simulink model "MCHP_SMO_MCLV48V300W_dsPIC33CK256MP508_DIM"  (R2022b)
settings: Solver=FixedStepDiscrete  StartTime=0.0  StopTime=10.0  FixedStep=50e-6  RelTol=1e-3  EnableMultiTasking=on
values from neighbouring files (symbols this model uses):
  Iq_Ref_openLoop = 1.5    [mcb_pmsm_foc_SMO_dsPIC33_data.m]
  PI_params = mcb.internal.SetControllerParameters(pmsm,inverter,PU_System,T_pwm,Ts,Ts_speed)    [mcb_pmsm_foc_SMO_dsPIC33_data.m]
  PU_System = mcb_SetPUSystem(pmsm,inverter)    [mcb_pmsm_foc_SMO_dsPIC33_data.m]
  PWM_frequency = 20e3    (= 20000)    [mcb_pmsm_foc_SMO_dsPIC33_data.m]
  Speed_Ref_openLoop = 700    [mcb_pmsm_foc_SMO_dsPIC33_data.m]
  Ts = T_pwm    (= 5e-05)    [mcb_pmsm_foc_SMO_dsPIC33_data.m]
  Ts_speed = 30*Ts    (= 0.0015)    [mcb_pmsm_foc_SMO_dsPIC33_data.m]
undefined symbols (not defined in the file or in its folder): A0, A4, AN0, AN1, B0, B2, C10, C11, C4, C5, D13, D14, D2, DiscIntNeverNeededParam, inverter, Max, MaxPer, ms, NumBits1, NumBits2, P20, P32, P52, P53, P58, P59, P66, P77, P78, Pin, pmsm, PWM1max, Resol, s, us
libraries: simulink x30, MCHP_Blockset x19, mcbcontrolslib x9, slpidlib x3, mcbplantlib x1, autolibpmsmexterior x1
(part 4 of 4)

== system MCHP_SMO_MCLV48V300W_dsPIC33CK256MP508_DIM/Current Control/Position and Speed Estimation1/Openloop Pos_PU ==
  Reset : ResetPort  DisableCoverage=on
  Constant : Constant  Value=Speed_Ref_openLoop/PU_System.N_base  OutDataTypeStr=dataType
  Data Type Conversion : DataTypeConversion  OutDataTypeStr=fixdt(1,32,20)  ConvertRealWorld=Stored Integer (SI)  SaturateOnIntegerOverflow=off  RndMeth=Floor
  Discrete-Time Integrator : DiscreteIntegrator  IntegratorMethod=Accumulation: Forward Euler  gainval=0.002  SampleTime=Ts  OutDataTypeStr=fixdt(1,32,20)  LimitOutput=on  UpperSaturationLimit=Speed_Ref_openLoop/PU_System.N_base  LowerSaturationLimit=0  ICPrevOutput=DiscIntNeverNeededParam  ICPrevScaledInput=DiscIntNeverNeededParam
  Gain : Gain  Gain=Ts*PU_System.N_base*pmsm.p/60  OutDataTypeStr=dataType  ParamDataTypeStr=Inherit: Same as input
  Position Generator : mcbcontrolslib/Position Generator  AngleOutput=Per-unit  ThetaSource=External  ThetaInput=5e-4  DataType=double  ExternalReset=none  Offset=0
  eps : Outport
  wires:
  Constant/1 -> Data Type Conversion/1
  Data Type Conversion/1 -> Discrete-Time Integrator/1
  Discrete-Time Integrator/1 -> Gain/1
  Position Generator/1 -> eps/1
  Gain/1 -> Position Generator/1

== system MCHP_SMO_MCLV48V300W_dsPIC33CK256MP508_DIM/Current Control/Position and Speed Estimation1/OpentoClosed ==
  Speed_fb : Inport
  Chart : Stateflow chart  TreatAsAtomicUnit=on
  Data Store Read5 : DataStoreRead  DataStoreName=Enable  IndexOptions=Index vector (dialog)  Indices=1  OutputSizes=1
  Data Store Write2 : DataStoreWrite  DataStoreName=EnableClosedLoop  IndexOptions=Index vector (dialog)  Indices=1  OutputSizes=1
  Data Type Conversion : DataTypeConversion  OutDataTypeStr=boolean  RndMeth=Simplest  SaturateOnIntegerOverflow=off
  Enable Closed Loop : Constant  OutDataTypeStr=uint16
  Enable Closed Loop1 : Constant  Value=Speed_Ref_openLoop/PU_System.N_base  OutDataTypeStr=dataType
  Open Loop Start-up : Constant  Value=0  OutDataTypeStr=uint16
  Switch2 : Switch  Criteria=u2 > Threshold  Threshold=1  SaturateOnIntegerOverflow=off  InputSameDT=off
  Terminator : Terminator
  EnClosedLoop : Outport
  wires:
  Open Loop Start-up/1 -> Switch2/3
  Data Store Read5/1 -> Chart/3(En)
  Chart/1(Mode) -> Switch2/2
  Switch2/1 -> Data Type Conversion/1
  Speed_fb/1 -> Chart/2(SpeedFb)
  Enable Closed Loop/1 -> Switch2/1
  Enable Closed Loop1/1 -> Chart/1(Limit)
  Chart/2(SpeedCtrl) -> Terminator/1
  Data Type Conversion/1 -> EnClosedLoop/1, Data Store Write2/1

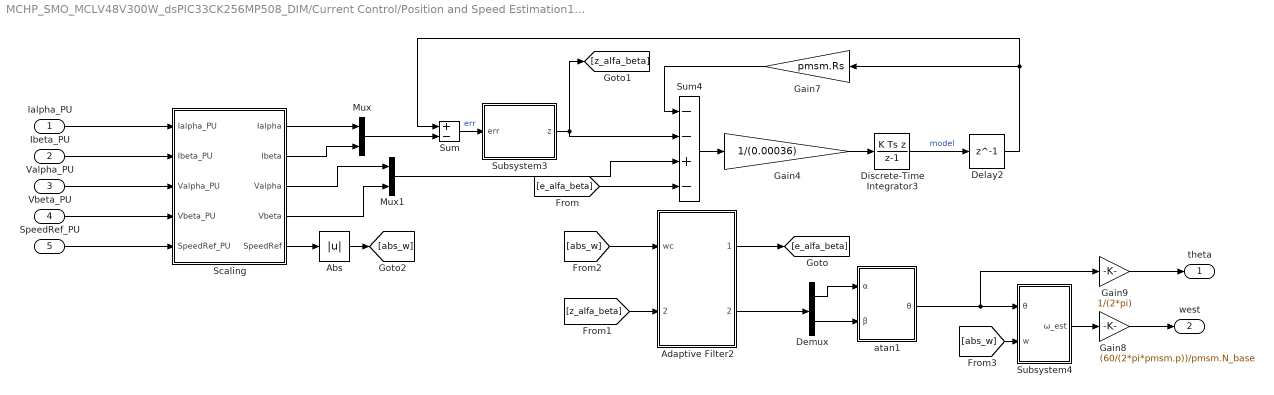
== system MCHP_SMO_MCLV48V300W_dsPIC33CK256MP508_DIM/Current Control/Position and Speed Estimation1/Sliding Mode Observer1 ==
  Ialpha_PU : Inport
  Ibeta_PU : Inport  Port=2
  Valpha_PU : Inport  Port=3
  Vbeta_PU : Inport  Port=4
  SpeedRef_PU : Inport  Port=5
  Abs : Abs  SaturateOnIntegerOverflow=off
  Adaptive Filter2 : Subsystem
  Delay2 : Delay  DelayLength=1
  Demux : Demux  Outputs=2
  Discrete-Time Integrator3 : DiscreteIntegrator  IntegratorMethod=Integration: Backward Euler  SampleTime=-1  OutDataTypeStr=Typecast_ci  ICPrevOutput=DiscIntNeverNeededParam  ICPrevScaledInput=DiscIntNeverNeededParam
  Gain4 : Gain  Gain=1/(0.00036)  OutDataTypeStr=fixdt(1,32,11)
  Gain7 : Gain  Gain=pmsm.Rs  OutDataTypeStr=Inherit: Same as input
  Gain8 : Gain  Gain=(60/(2*pi*pmsm.p))/pmsm.N_base  OutDataTypeStr=dataType
  Gain9 : Gain  Gain=1/(2*pi)  OutDataTypeStr=dataType
  Mux : Mux  Inputs=2
  Mux1 : Mux  Inputs=2
  Scaling : Subsystem
  Subsystem3 : Subsystem
  Subsystem4 : Subsystem
  Sum : Sum  Inputs=+-  AccumDataTypeStr=Typecast_ci  OutDataTypeStr=Typecast_ci
  Sum4 : Sum  Inputs=--+-  AccumDataTypeStr=Typecast_di  OutDataTypeStr=Typecast_di
  atan1 : Subsystem
  theta : Outport
  west : Outport  Port=2
  wires:
  Ialpha_PU/1 -> Scaling/1(Ialpha_PU)
  Vbeta_PU/1 -> Scaling/4(Vbeta_PU)
  Valpha_PU/1 -> Scaling/3(Valpha_PU)
  Ibeta_PU/1 -> Scaling/2(Ibeta_PU)
  SpeedRef_PU/1 -> Scaling/5(SpeedRef_PU)
  Gain7/1 -> Sum4/1
  Discrete-Time Integrator3/1 -> Delay2/1  "model"
  atan1/1(θ) -> Gain9/1, Subsystem4/1(θ)
  Sum4/1 -> Gain4/1
  Mux1/1 -> Sum4/3
  Gain4/1 -> Discrete-Time Integrator3/1
  Subsystem4/1(ω_est) -> Gain8/1
  Subsystem3/1(z) -> [z_alfa_beta], Sum4/2
  Gain9/1 -> theta/1
  Gain8/1 -> west/1
  Sum/1 -> Subsystem3/1(err)  "err"
  Scaling/5(SpeedRef) -> Abs/1
  Scaling/1(Ialpha) -> Mux/1
  Scaling/2(Ibeta) -> Mux/2
  Scaling/3(Valpha) -> Mux1/1
  Scaling/4(Vbeta) -> Mux1/2
  [e_alfa_beta] -> Sum4/4
  Mux/1 -> Sum/2
  Delay2/1 -> Sum/1, Gain7/1
  Adaptive Filter2/1(ealfa_bita) -> [e_alfa_beta]
  Adaptive Filter2/2(ealfa_bita_fil) -> Demux/1
  [z_alfa_beta] -> Adaptive Filter2/2(zalfa_bita)
  Abs/1 -> [abs_w]
  [abs_w] -> Adaptive Filter2/1(wc)
  Demux/1 -> atan1/1(α)
  Demux/2 -> atan1/2(β)
  [abs_w] -> Subsystem4/2(w)

== system MCHP_SMO_MCLV48V300W_dsPIC33CK256MP508_DIM/Current Control/Serial Tx/UART_TX ==
  Count : Inport
  Data : Inport  Port=2
  Debug_Data : Subsystem
  SCI_Tx : Subsystem
  wires:
  Count/1 -> Debug_Data/1(Count)
  Debug_Data/1(Data_log) -> SCI_Tx/1(Data_Log)
  Data/1 -> Debug_Data/2(Data)

== system MCHP_SMO_MCLV48V300W_dsPIC33CK256MP508_DIM/Inverter and Motor/Simulation/Inverter ==
  Duty_abc : Inport
  Average-Value Inverter : mcbplantlib/Average-Value Inverter
  Constant2 : Constant  Value=inverter.V_dc  OutDataTypeStr=single  SampleTime=-1
  Data Type Conversion1 : DataTypeConversion  OutDataTypeStr=single  RndMeth=Simplest  SaturateOnIntegerOverflow=off
  Vabc : Outport  VectorParamsAs1DForOutWhenUnconnected=off
  wires:
  Average-Value Inverter/1 -> Vabc/1
  Data Type Conversion1/1 -> Average-Value Inverter/1
  Duty_abc/1 -> Data Type Conversion1/1
  Constant2/1 -> Average-Value Inverter/2

== system MCHP_SMO_MCLV48V300W_dsPIC33CK256MP508_DIM/Inverter and Motor/Simulation/Load_Profile (Torque) ==
  Data Type Conversion : DataTypeConversion  OutDataTypeStr=single  SaturateOnIntegerOverflow=off  RndMeth=Floor
  IIR Filter : mcbcontrolslib/IIR Filter  VariantControl=Low Pass Filter  VariantSelect=Low-pass  Filter_constant=0.01  advancedSettings=off  Ts=50e-6  cutOff_freq=32.1525
  Rate Limiter1 : RateLimiter  RisingSlewLimit=0.5  FallingSlewLimit=-0.2  SampleTimeMode=inherited
  Step : Step  Time=5  Before=0.0* pmsm.T_rated  After=0.25* pmsm.T_rated
  Step1 : Step  Time=8  Before=0.25* pmsm.T_rated  After=0.7*pmsm.T_rated
  Step2 : Step  Time=8  Before=1  After=0
  Switch : Switch  Criteria=u2 > Threshold  SaturateOnIntegerOverflow=off  InputSameDT=off
  Load_Trq : Outport  VectorParamsAs1DForOutWhenUnconnected=off
  wires:
  IIR Filter/1 -> Load_Trq/1
  Data Type Conversion/1 -> IIR Filter/1
  Switch/1 -> Rate Limiter1/1
  Step1/1 -> Switch/3
  Step/1 -> Switch/1
  Step2/1 -> Switch/2
  Rate Limiter1/1 -> Data Type Conversion/1

== system MCHP_SMO_MCLV48V300W_dsPIC33CK256MP508_DIM/Inverter and Motor/Simulation/Sensor_Measurements ==
  PhaseCurr : Inport
  Data Type Conversion4 : DataTypeConversion  OutDataTypeStr=single  RndMeth=Simplest  SaturateOnIntegerOverflow=off
  Delay1 : Delay  DelayLength=PI_params.delay_Currents
  Inverting OpAmp : Gain  Gain=1/PU_System.I_base  OutDataTypeStr=dataType  RndMeth=Simplest
  Selector : Selector  InputPortWidth=3  IndexOptions=Index vector (dialog)  Indices=[1 2]  OutputSizes=1
  Iab_fb : Outport  VectorParamsAs1DForOutWhenUnconnected=off
  wires:
  Selector/1 -> Inverting OpAmp/1
  PhaseCurr/1 -> Data Type Conversion4/1
  Data Type Conversion4/1 -> Delay1/1
  Delay1/1 -> Selector/1  "Iab_fb"
  Inverting OpAmp/1 -> Iab_fb/1

== system MCHP_SMO_MCLV48V300W_dsPIC33CK256MP508_DIM/Speed Control/Enable Switch/Codegen ==

== system MCHP_SMO_MCLV48V300W_dsPIC33CK256MP508_DIM/Speed Control/Enable Switch/Sim ==
  Constant : Constant  OutDataTypeStr=Inherit: Inherit via back propagation
  Data Store Write : DataStoreWrite  DataStoreName=Enable  IndexOptions=Index vector (dialog)  Indices=1  OutputSizes=1
  wires:
  Constant/1 -> Data Store Write/1

== system MCHP_SMO_MCLV48V300W_dsPIC33CK256MP508_DIM/Current Control/Closed Loop Control1/Current_Controllers/PI_Controller_Id ==
  I_ref : Inport
  I_fb : Inport  Port=2
  AND : Logic  IconShape=distinctive  AllPortsSameDT=off  OutDataTypeStr=boolean
  Data Store Read : DataStoreRead  DataStoreName=Enable  IndexOptions=Index vector (dialog)  Indices=1  OutputSizes=1
  Data Store Read1 : DataStoreRead  DataStoreName=EnableFOC  IndexOptions=Index vector (dialog)  Indices=1  OutputSizes=1
  Discrete PI Controller with anti-windup & reset : slpidlib/PID Controller  Controller=PI  Form=Parallel  TimeDomain=Discrete-time  UseExternalTs=off  SampleTime=-1  IntegratorMethod=Forward Euler  FilterMethod=Forward Euler  ControllerParametersSource=external  P=1  I=1  UseKiTs=on  D=0  N=100  UseFilter=on  TunerSelectOption=Transfer Function Based (PID Tuner App)  InitialConditionSource=external  InitialConditionForIntegrator=0  InitialConditionForFilter=0  DifferentiatorICPrevScaledInput=0  ExternalReset=level  TrackingMode=off  Kt=1  LimitOutput=on  SatLimitsSource=internal  UpperSaturationLimit=1  LowerSaturationLimit=-1  LinearizeAsGain=on  AntiWindupMode=clamping  Kb=1  LimitIntegrator=off  UpperIntegratorSaturationLimit=inf  LowerIntegratorSaturationLimit=-inf  RndMeth=Simplest  POutMin=[]  POutMax=[]  IOutMin=[]  IOutMax=[]  DOutMin=[]  DOutMax=[]  NOutMin=[]  NOutMax=[]  SumOutMin=[]  SumOutMax=[]  SaturationOutDataTypeStr=Inherit: Inherit via back propagation  SaturationOutMin=[]  SaturationOutMax=[]  PParamMin=[]  PParamMax=[]  IParamMin=[]  IParamMax=[]  DParamMin=[]  DParamMax=[]  NParamMin=[]  NParamMax=[]  KbParamMin=[]  KbParamMax=[]  KtParamMin=[]  KtParamMax=[]  KbOutMin=[]  KbOutMax=[]  KtOutMin=[]  KtOutMax=[]  IntegratorOutMin=[]  IntegratorOutMax=[]  FilterOutMin=[]  FilterOutMax=[]  SumI1OutMin=[]  SumI1OutMax=[]  SumI2OutMin=[]  SumI2OutMax=[]  SumI3OutMin=[]  SumI3OutMax=[]  SumI4OutMin=[]  SumI4OutMax=[]  SumDOutMin=[]  SumDOutMax=[]  DifferentiatorOutMin=[]  DifferentiatorOutMax=[]  FilterDiffOutCoefMin=[]  FilterDiffOutCoefMax=[]  ReciprocalOutMin=[]  ReciprocalOutMax=[]  SumDenOutMin=[]  SumDenOutMax=[]  SumNumOutMin=[]  SumNumOutMax=[]  DivideOutMin=[]  DivideOutMax=[]  UdiffTsProdOutMin=[]  UdiffTsProdOutMax=[]  NTsProdOutMin=[]  NTsProdOutMax=[]  UintegralTsProdOutMin=[]  UintegralTsProdOutMax=[]  UngainTsProdOutMin=[]  UngainTsProdOutMax=[]  ClampingZeroOutDataTypeStr=Inherit: Inherit via back propagation  ClampingZeroOutMin=[]  ClampingZeroOutMax=[]  FilterDenConstantOutDataTypeStr=Inherit: Inherit via back propagation  FilterDenConstantOutMin=[]  FilterDenConstantOutMax=[]  PCopyOutDataTypeStr=Inherit: Inherit via back propagation  PCopyOutMin=[]  PCopyOutMax=[]  NCopyOutDataTypeStr=Inherit: Inherit via back propagation  NCopyOutMin=[]  NCopyOutMax=[]  IntegratorContinuousStateAttributes=''  IntegratorStateMustResolveToSignalObject=off  IntegratorRTWStateStorageClass=Auto  FilterContinuousStateAttributes=''  FilterStateMustResolveToSignalObject=off  FilterRTWStateStorageClass=Auto  ParallelPVariant=ExternalParameters  IdealPVariant=Disabled  IVariant=ExternalParameters  DVariant=Disabled  IntegratorVariant=Discrete  SatVariant=Enabled  AWVariant=DiscClampingParallel  PCopyVariant=Disabled  TRVariant=Disabled  FdbkBlocksVariant=Forward  IdealPFdbkVariant=Disabled  SatFdbkVariant=Disabled  DerivativeFilterVariant=Disabled  NVariant=Disabled  NCopyVariant=Disabled_SignalSpec  FilterICVariant=Disabled  IntegratorICVariant=ExternalICs  ExternalResetVariant=ExternalReset  TRSumVariant=Passthrough  SumFdbkVariant=Disabled  SumVariant=Sum_PI  TsampFilterVariant=InternalTs  TsampNgainVariant=Passthrough  TsampIntegralVariant=Passthrough  ExternalSaturationOutDataTypeStr=Inherit: Same as second input
  Ki : Constant  Value=PI_params.Ki_i*Ts/2  OutDataTypeStr=dataType  SampleTime=-1
  Ki1 : Constant  Value=0  OutDataTypeStr=dataType  SampleTime=-1
  Kp : Constant  Value=PI_params.Kp_i/2  OutDataTypeStr=dataType2  SampleTime=-1
  Logical Operator : Logic  Operator=NOT  IconShape=distinctive  AllPortsSameDT=off  OutDataTypeStr=boolean
  Sum : Sum  Inputs=|+-  OutDataTypeStr=Inherit: Same as first input
  V_ref : Outport  VectorParamsAs1DForOutWhenUnconnected=off
  wires:
  I_ref/1 -> Sum/1
  I_fb/1 -> Sum/2
  Data Store Read1/1 -> AND/1
  Discrete PI Controller with anti-windup & reset/1 -> V_ref/1
  Sum/1 -> Discrete PI Controller with anti-windup & reset/1
  Kp/1 -> Discrete PI Controller with anti-windup & reset/2
  Ki/1 -> Discrete PI Controller with anti-windup & reset/3
  Logical Operator/1 -> Discrete PI Controller with anti-windup & reset/4
  Ki1/1 -> Discrete PI Controller with anti-windup & reset/5
  Data Store Read/1 -> AND/2
  AND/1 -> Logical Operator/1

== system MCHP_SMO_MCLV48V300W_dsPIC33CK256MP508_DIM/Current Control/Closed Loop Control1/Current_Controllers/PI_Controller_Iq ==
  I_ref : Inport
  I_fb : Inport  Port=2
  AND : Logic  IconShape=distinctive  AllPortsSameDT=off  OutDataTypeStr=boolean
  Data Store Read : DataStoreRead  DataStoreName=Enable  IndexOptions=Index vector (dialog)  Indices=1  OutputSizes=1
  Data Store Read1 : DataStoreRead  DataStoreName=EnableFOC  IndexOptions=Index vector (dialog)  Indices=1  OutputSizes=1
  Discrete PI Controller with anti-windup & reset : slpidlib/PID Controller  Controller=PI  Form=Parallel  TimeDomain=Discrete-time  UseExternalTs=off  SampleTime=-1  IntegratorMethod=Forward Euler  FilterMethod=Forward Euler  ControllerParametersSource=external  P=1  I=1  UseKiTs=on  D=0  N=100  UseFilter=on  TunerSelectOption=Transfer Function Based (PID Tuner App)  InitialConditionSource=external  InitialConditionForIntegrator=0  InitialConditionForFilter=0  DifferentiatorICPrevScaledInput=0  ExternalReset=level  TrackingMode=off  Kt=1  LimitOutput=on  SatLimitsSource=internal  UpperSaturationLimit=1  LowerSaturationLimit=-1  LinearizeAsGain=on  AntiWindupMode=clamping  Kb=1  LimitIntegrator=off  UpperIntegratorSaturationLimit=inf  LowerIntegratorSaturationLimit=-inf  RndMeth=Simplest  POutMin=[]  POutMax=[]  IOutMin=[]  IOutMax=[]  DOutMin=[]  DOutMax=[]  NOutMin=[]  NOutMax=[]  SumOutMin=[]  SumOutMax=[]  SaturationOutDataTypeStr=Inherit: Inherit via back propagation  SaturationOutMin=[]  SaturationOutMax=[]  PParamMin=[]  PParamMax=[]  IParamMin=[]  IParamMax=[]  DParamMin=[]  DParamMax=[]  NParamMin=[]  NParamMax=[]  KbParamMin=[]  KbParamMax=[]  KtParamMin=[]  KtParamMax=[]  KbOutMin=[]  KbOutMax=[]  KtOutMin=[]  KtOutMax=[]  IntegratorOutMin=[]  IntegratorOutMax=[]  FilterOutMin=[]  FilterOutMax=[]  SumI1OutMin=[]  SumI1OutMax=[]  SumI2OutMin=[]  SumI2OutMax=[]  SumI3OutMin=[]  SumI3OutMax=[]  SumI4OutMin=[]  SumI4OutMax=[]  SumDOutMin=[]  SumDOutMax=[]  DifferentiatorOutMin=[]  DifferentiatorOutMax=[]  FilterDiffOutCoefMin=[]  FilterDiffOutCoefMax=[]  ReciprocalOutMin=[]  ReciprocalOutMax=[]  SumDenOutMin=[]  SumDenOutMax=[]  SumNumOutMin=[]  SumNumOutMax=[]  DivideOutMin=[]  DivideOutMax=[]  UdiffTsProdOutMin=[]  UdiffTsProdOutMax=[]  NTsProdOutMin=[]  NTsProdOutMax=[]  UintegralTsProdOutMin=[]  UintegralTsProdOutMax=[]  UngainTsProdOutMin=[]  UngainTsProdOutMax=[]  ClampingZeroOutDataTypeStr=Inherit: Inherit via back propagation  ClampingZeroOutMin=[]  ClampingZeroOutMax=[]  FilterDenConstantOutDataTypeStr=Inherit: Inherit via back propagation  FilterDenConstantOutMin=[]  FilterDenConstantOutMax=[]  PCopyOutDataTypeStr=Inherit: Inherit via back propagation  PCopyOutMin=[]  PCopyOutMax=[]  NCopyOutDataTypeStr=Inherit: Inherit via back propagation  NCopyOutMin=[]  NCopyOutMax=[]  IntegratorContinuousStateAttributes=''  IntegratorStateMustResolveToSignalObject=off  IntegratorRTWStateStorageClass=Auto  FilterContinuousStateAttributes=''  FilterStateMustResolveToSignalObject=off  FilterRTWStateStorageClass=Auto  ParallelPVariant=ExternalParameters  IdealPVariant=Disabled  IVariant=ExternalParameters  DVariant=Disabled  IntegratorVariant=Discrete  SatVariant=Enabled  AWVariant=DiscClampingParallel  PCopyVariant=Disabled  TRVariant=Disabled  FdbkBlocksVariant=Forward  IdealPFdbkVariant=Disabled  SatFdbkVariant=Disabled  DerivativeFilterVariant=Disabled  NVariant=Disabled  NCopyVariant=Disabled_SignalSpec  FilterICVariant=Disabled  IntegratorICVariant=ExternalICs  ExternalResetVariant=ExternalReset  TRSumVariant=Passthrough  SumFdbkVariant=Disabled  SumVariant=Sum_PI  TsampFilterVariant=InternalTs  TsampNgainVariant=Passthrough  TsampIntegralVariant=Passthrough  ExternalSaturationOutDataTypeStr=Inherit: Same as second input
  Ki : Constant  Value=PI_params.Ki_i*Ts/2  OutDataTypeStr=dataType  SampleTime=-1
  Kp : Constant  Value=PI_params.Kp_i/2  OutDataTypeStr=dataType2  SampleTime=-1
  Kp1 : Constant  Value=0  OutDataTypeStr=dataType  SampleTime=-1
  Logical Operator : Logic  Operator=NOT  IconShape=distinctive  AllPortsSameDT=off  OutDataTypeStr=boolean
  Sum : Sum  Inputs=|+-  OutDataTypeStr=Inherit: Same as first input
  V_ref : Outport  VectorParamsAs1DForOutWhenUnconnected=off
  wires:
  Discrete PI Controller with anti-windup & reset/1 -> V_ref/1
  Data Store Read1/1 -> AND/1
  I_fb/1 -> Sum/2
  I_ref/1 -> Sum/1
  Kp/1 -> Discrete PI Controller with anti-windup & reset/2
  Sum/1 -> Discrete PI Controller with anti-windup & reset/1
  Ki/1 -> Discrete PI Controller with anti-windup & reset/3
  Logical Operator/1 -> Discrete PI Controller with anti-windup & reset/4
  Kp1/1 -> Discrete PI Controller with anti-windup & reset/5
  Data Store Read/1 -> AND/2
  AND/1 -> Logical Operator/1

== system MCHP_SMO_MCLV48V300W_dsPIC33CK256MP508_DIM/Current Control/Output Scaling/Mode Selector/Subsystem1 ==
  Count : Inport
  AND : Logic  IconShape=distinctive  AllPortsSameDT=off  OutDataTypeStr=boolean
  Compare To Constant : simulink/Logic and Bit Operations/Compare To Constant  relop=>=  const=2  OutDataTypeStr=boolean
  Compare To Constant1 : simulink/Logic and Bit Operations/Compare To Constant  relop=<  const=1  OutDataTypeStr=boolean
  Compare To Constant2 : simulink/Logic and Bit Operations/Compare To Constant  relop=<  const=2  OutDataTypeStr=boolean
  Compare To Constant3 : simulink/Logic and Bit Operations/Compare To Constant  relop=>  const=1  OutDataTypeStr=boolean
  Data Store Write : DataStoreWrite  DataStoreName=EnCurOffset  IndexOptions=Index vector (dialog)  Indices=1  OutputSizes=1
  Data Store Write1 : DataStoreWrite  DataStoreName=EnableFOC  IndexOptions=Index vector (dialog)  Indices=1  OutputSizes=1
  Gain : Gain  Gain=1/PWM_frequency  OutDataTypeStr=dataType2  RndMeth=Simplest
  Current Offset : Outport
  PositionOffset : Outport  Port=2
  EnableFOC : Outport  Port=3
  wires:
  Count/1 -> Gain/1
  Gain/1 -> Compare To Constant1/1, Compare To Constant3/1, Compare To Constant2/1, Compare To Constant/1
  Compare To Constant1/1 -> Data Store Write/1, Current Offset/1
  Compare To Constant2/1 -> AND/2
  Compare To Constant3/1 -> AND/1
  AND/1 -> PositionOffset/1
  Compare To Constant/1 -> Data Store Write1/1, EnableFOC/1

== system MCHP_SMO_MCLV48V300W_dsPIC33CK256MP508_DIM/Current Control/Output Scaling/Mode Selector/Up Counter ==
  Enable : EnablePort  StatesWhenEnabling=reset
  Add1 : Sum  SaturateOnIntegerOverflow=on
  Constant : Constant  OutDataTypeStr=uint32
  Delay : Delay  DelayLength=1
  Count : Outport  InitialOutput=0
  wires:
  Delay/1 -> Add1/2
  Add1/1 -> Count/1, Delay/1
  Constant/1 -> Add1/1

== system MCHP_SMO_MCLV48V300W_dsPIC33CK256MP508_DIM/Current Control/Position and Speed Estimation1/Sliding Mode Observer1/Adaptive Filter2 ==
  wc : Inport
  zalfa_bita : Inport  Port=2
  Delay : Delay  DelayLength=1
  Delay3 : Delay  DelayLength=1
  Discrete-Time Integrator : DiscreteIntegrator  IntegratorMethod=Integration: Backward Euler  SampleTime=-1  OutDataTypeStr=Typecast_BEMF  ICPrevOutput=DiscIntNeverNeededParam  ICPrevScaledInput=DiscIntNeverNeededParam
  Discrete-Time Integrator2 : DiscreteIntegrator  IntegratorMethod=Integration: Backward Euler  SampleTime=-1  OutDataTypeStr=Typecast_BEMF  ICPrevOutput=DiscIntNeverNeededParam  ICPrevScaledInput=DiscIntNeverNeededParam
  Product : Product  OutDataTypeStr=fixdt(1,32,8)
  Product2 : Product  OutDataTypeStr=fixdt(1,32,8)
  Sum2 : Sum  Inputs=|+-  OutDataTypeStr=Inherit: Same as first input
  Sum3 : Sum  Inputs=|+-  AccumDataTypeStr=fixdt(1,16,8)  OutDataTypeStr=fixdt(1,16,8)
  ealfa_bita : Outport  VectorParamsAs1DForOutWhenUnconnected=off
  ealfa_bita_fil : Outport  Port=2  VectorParamsAs1DForOutWhenUnconnected=off
  wires:
  Sum2/1 -> Product/2
  Product/1 -> Discrete-Time Integrator/1
  Product2/1 -> Discrete-Time Integrator2/1
  Sum3/1 -> Product2/2
  zalfa_bita/1 -> Sum2/1
  Delay/1 -> Sum2/2
  Delay3/1 -> Sum3/2
  wc/1 -> Product/1, Product2/1
  Discrete-Time Integrator2/1 -> ealfa_bita_fil/1, Delay3/1
  Discrete-Time Integrator/1 -> Delay/1, ealfa_bita/1, Sum3/1

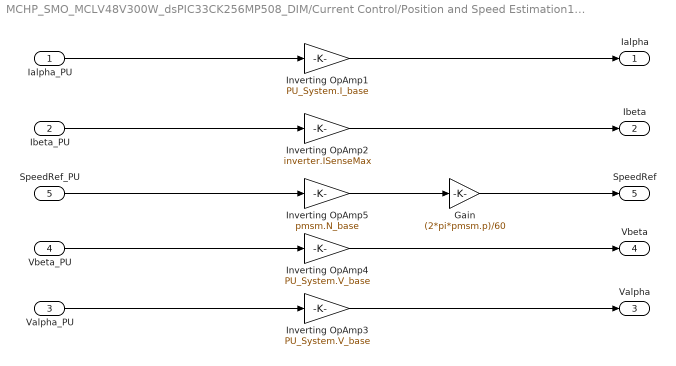
== system MCHP_SMO_MCLV48V300W_dsPIC33CK256MP508_DIM/Current Control/Position and Speed Estimation1/Sliding Mode Observer1/Scaling ==
  Ialpha_PU : Inport
  Ibeta_PU : Inport  Port=2
  Valpha_PU : Inport  Port=3
  Vbeta_PU : Inport  Port=4
  SpeedRef_PU : Inport  Port=5
  Gain : Gain  Gain=(2*pi*pmsm.p)/60  OutDataTypeStr=fixdt(1,16,3)
  Inverting OpAmp1 : Gain  Gain=PU_System.I_base  OutDataTypeStr=fixdt(1,16,11)  RndMeth=Simplest
  Inverting OpAmp2 : Gain  Gain=inverter.ISenseMax  OutDataTypeStr=fixdt(1,16,11)  RndMeth=Simplest
  Inverting OpAmp3 : Gain  Gain=PU_System.V_base  OutDataTypeStr=fixdt(1,16,11)  RndMeth=Simplest
  Inverting OpAmp4 : Gain  Gain=PU_System.V_base  OutDataTypeStr=fixdt(1,16,11)  RndMeth=Simplest
  Inverting OpAmp5 : Gain  Gain=pmsm.N_base  OutDataTypeStr=fixdt(1,16,2)  RndMeth=Simplest
  Ialpha : Outport
  Ibeta : Outport  Port=2
  Valpha : Outport  Port=3
  Vbeta : Outport  Port=4
  SpeedRef : Outport  Port=5
  wires:
  Vbeta_PU/1 -> Inverting OpAmp4/1
  SpeedRef_PU/1 -> Inverting OpAmp5/1
  Inverting OpAmp2/1 -> Ibeta/1
  Inverting OpAmp3/1 -> Valpha/1
  Ibeta_PU/1 -> Inverting OpAmp2/1
  Inverting OpAmp4/1 -> Vbeta/1
  Ialpha_PU/1 -> Inverting OpAmp1/1
  Inverting OpAmp1/1 -> Ialpha/1
  Valpha_PU/1 -> Inverting OpAmp3/1
  Inverting OpAmp5/1 -> Gain/1
  Gain/1 -> SpeedRef/1

== system MCHP_SMO_MCLV48V300W_dsPIC33CK256MP508_DIM/Current Control/Position and Speed Estimation1/Sliding Mode Observer1/Subsystem3 ==
  err : Inport
  Abs1 : Abs  SaturateOnIntegerOverflow=off
  Compare To Constant1 : simulink/Logic and Bit Operations/Compare To Constant  relop=>=  const=1.0303  OutDataTypeStr=boolean
  Gain4 : Gain  Gain=7.5512  OutDataTypeStr=Typecast_BEMF
  Gain7 : Gain  Gain=7.7800  OutDataTypeStr=Typecast_BEMF
  Sign1 : Signum
  Switch1 : Switch  Criteria=u2 > Threshold  SaturateOnIntegerOverflow=off  InputSameDT=off  OutDataTypeStr=Inherit: Same as first input
  z : Outport
  wires:
  Switch1/1 -> z/1
  Gain4/1 -> Switch1/3  "z"
  Abs1/1 -> Compare To Constant1/1
  Gain7/1 -> Switch1/1
  Compare To Constant1/1 -> Switch1/2
  err/1 -> Gain4/1, Abs1/1, Sign1/1
  Sign1/1 -> Gain7/1  "z"

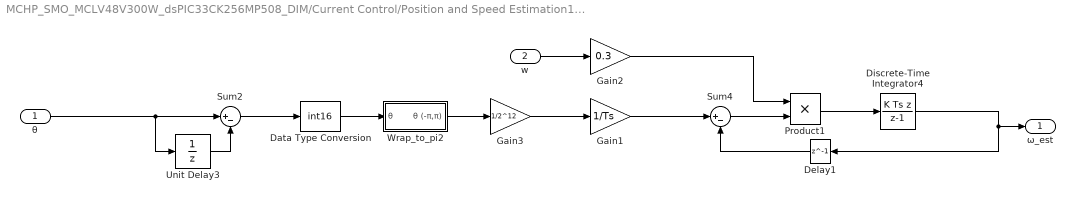
== system MCHP_SMO_MCLV48V300W_dsPIC33CK256MP508_DIM/Current Control/Position and Speed Estimation1/Sliding Mode Observer1/Subsystem4 ==
  θ : Inport
  w : Inport  Port=2
  Data Type Conversion : DataTypeConversion  OutDataTypeStr=int16  ConvertRealWorld=Stored Integer (SI)  SaturateOnIntegerOverflow=off  RndMeth=Floor
  Delay1 : Delay  DelayLength=1
  Discrete-Time Integrator4 : DiscreteIntegrator  IntegratorMethod=Integration: Backward Euler  SampleTime=-1  OutDataTypeStr=fixdt(1,16,3)  ICPrevOutput=DiscIntNeverNeededParam  ICPrevScaledInput=DiscIntNeverNeededParam
  Gain1 : Gain  Gain=1/Ts  OutDataTypeStr=fixdt(1,16,3)
  Gain2 : Gain  Gain=0.3  OutDataTypeStr=fixdt(1,16,3)
  Gain3 : Gain  Gain=1/2^12  OutDataTypeStr=fixdt(1,16,12)
  Product1 : Product  OutDataTypeStr=fixdt(1,32,8)
  Sum2 : Sum  Inputs=|+-  AccumDataTypeStr=fixdt(1,16,12)  OutDataTypeStr=fixdt(1,16,12)
  Sum4 : Sum  Inputs=|+-  OutDataTypeStr=Inherit: Same as first input
  Unit Delay3 : UnitDelay  SampleTime=Ts  HasFrameUpgradeWarning=on
  Wrap_to_pi2 : Subsystem  VariantControl=VSS_STD
  ω_est : Outport  VectorParamsAs1DForOutWhenUnconnected=off
  wires:
  Unit Delay3/1 -> Sum2/2
  θ/1 -> Sum2/1, Unit Delay3/1
  Wrap_to_pi2/1(θ (-π,π)) -> Gain3/1
  Sum4/1 -> Product1/2
  Product1/1 -> Discrete-Time Integrator4/1
  Delay1/1 -> Sum4/2
  Sum2/1 -> Data Type Conversion/1
  Data Type Conversion/1 -> Wrap_to_pi2/1(θ)
  Gain3/1 -> Gain1/1
  Gain1/1 -> Sum4/1
  Discrete-Time Integrator4/1 -> ω_est/1, Delay1/1
  w/1 -> Gain2/1
  Gain2/1 -> Product1/1

== system MCHP_SMO_MCLV48V300W_dsPIC33CK256MP508_DIM/Current Control/Position and Speed Estimation1/Sliding Mode Observer1/atan1 ==
  note: Consistent with Microchip notation:
      |
      | x_α = cos(θ) * x_d - sin(θ) * x_q
      | x_β = sin(θ) * x_d + cos(θ) * x_q
      |
      | θ = atan2(sin(θ)/cos(θ)) = atan2(-x_α/x_β)
      |
      | provided x_d = 0, which is true in case of E_d
  α : Inport
  β : Inport  Port=2
  Bias3 : Bias  Bias=1.244/(2*pi)  SaturateOnIntegerOverflow=off
  Cast2 : DataTypeConversion  OutDataTypeStr=fixdt(0,16,16)  ConvertRealWorld=Stored Integer (SI)  SaturateOnIntegerOverflow=off  RndMeth=Floor
  Gain3 : Gain  Gain=-1  OutDataTypeStr=Inherit: Same as input
  Gain5 : Gain  Gain=2*pi  OutDataTypeStr=fixdt(1,16,12)
  Trigonometric Function1 : Trigonometry  Operator=atan2  ApproximationMethod=Lookup  AngleUnit=revolution  TableDataTypeStr=fixdt(1,16,16)
  θ : Outport  VectorParamsAs1DForOutWhenUnconnected=off
  wires:
  α/1 -> Gain3/1
  β/1 -> Trigonometric Function1/2
  Trigonometric Function1/1 -> Cast2/1
  Gain3/1 -> Trigonometric Function1/1
  Cast2/1 -> Bias3/1
  Bias3/1 -> Gain5/1
  Gain5/1 -> θ/1

== system MCHP_SMO_MCLV48V300W_dsPIC33CK256MP508_DIM/Current Control/Serial Tx/UART_TX/Debug_Data ==
  Count : Inport
  Data : Inport  Port=2
  Bitwise Operator2 : simulink/Logic and Bit Operations/Bitwise Operator  logicop=AND  UseBitMask=on  BitMask=bin2dec('0000000011111111')  BitMaskRealWorld=Stored Integer
  Bitwise Operator3 : simulink/Logic and Bit Operations/Bitwise Operator  logicop=AND  UseBitMask=on  BitMask=bin2dec('0000000011111111')  BitMaskRealWorld=Stored Integer
  Data Type Conversion1 : DataTypeConversion  OutDataTypeStr=uint8  RndMeth=Simplest  SaturateOnIntegerOverflow=off
  Data Type Conversion2 : DataTypeConversion  OutDataTypeStr=uint8  RndMeth=Simplest  SaturateOnIntegerOverflow=off
  Data Type Conversion3 : DataTypeConversion  OutDataTypeStr=uint16  ConvertRealWorld=Stored Integer (SI)  RndMeth=Simplest  SaturateOnIntegerOverflow=off
  Mux : Mux  Inputs=3
  Shift Arithmetic2 : ArithShift  BitShiftNumber=8  BitShiftDirection=Right
  Data_log : Outport
  wires:
  Mux/1 -> Data_log/1
  Data/1 -> Data Type Conversion3/1
  Count/1 -> Mux/1
  Bitwise Operator2/1 -> Data Type Conversion1/1
  Shift Arithmetic2/1 -> Bitwise Operator3/1
  Bitwise Operator3/1 -> Data Type Conversion2/1
  Data Type Conversion3/1 -> Bitwise Operator2/1, Shift Arithmetic2/1
  Data Type Conversion1/1 -> Mux/2
  Data Type Conversion2/1 -> Mux/3

== system MCHP_SMO_MCLV48V300W_dsPIC33CK256MP508_DIM/Current Control/Serial Tx/UART_TX/SCI_Tx ==
  Data_Log : Inport
  End : Constant  Value=hex2dec('45')  OutDataTypeStr=uint8
  Mux : Mux  Inputs=3
  Start : Constant  Value=hex2dec('53')  OutDataTypeStr=uint8
  UART Tx : MCHP_Blockset/BUS UART/UART Tx  UART_REF=1  ORDERING=None  AllOrNothing=off  SampleTime=-1  MCHP_MASTERLINK=MCHP_SMO_MCLV48V300W_dsPIC33CK256MP508_DIM/BOARD MCLV-48V-300W dsPIC33CK256MP508 MC DIM/Microchip Master  NSend_Input=off  UART_String=off  NSend_Output=off
      settings: SourceProductName=MPLAB Device Blocks for Simulink
  wires:
  Mux/1 -> UART Tx/1
  Data_Log/1 -> Mux/2
  Start/1 -> Mux/1
  End/1 -> Mux/3

== system MCHP_SMO_MCLV48V300W_dsPIC33CK256MP508_DIM/Current Control/Position and Speed Estimation1/Sliding Mode Observer1/Subsystem4/Wrap_to_pi2 ==
  note: What's left after
      | division by 2pi
  note: This block limits the output angle between +/- π.
  note: Add pi
  note: What's left after
      | division by 2pi
      | again
  note: Subtract pi
  θ : Inport
  Bias : Bias  Bias=pi*4096  SaturateOnIntegerOverflow=off
  Bias1 : Bias  Bias=-pi*4096  SaturateOnIntegerOverflow=off
  Math Function : Math  Operator=mod  SignedPower=on
  Math Function1 : Math  Operator=mod  SignedPower=on
  load torque1 : Constant  Value=2*pi*4096  OutDataTypeStr=int16  SampleTime=Ts
  θ (-π,π) : Outport  VectorParamsAs1DForOutWhenUnconnected=off
  wires:
  Math Function1/1 -> Bias/1
  θ/1 -> Math Function1/1
  Math Function/1 -> Bias1/1
  load torque1/1 -> Math Function1/2, Math Function/2
  Bias/1 -> Math Function/1
  Bias1/1 -> θ (-π,π)/1

== stateflow chart MCHP_SMO_MCLV48V300W_dsPIC33CK256MP508_DIM/Current Control/Position and Speed Estimation1/OpentoClosed/Chart ==
  state Init
    during: Mode = 0;
    SpeedCtrl = 0;
  state Align
    during: Mode = 0;
    SpeedCtrl = 0;
  state ClosedLoopFilter
    during: Mode = 2;
    SpeedCtrl = 1;
  state ClosedLoop
    during: Mode = 2;
    SpeedCtrl = 0;
  state OpenLoop
    during: Mode = 1;
    SpeedCtrl = 0;
  (default) -> Init
  ClosedLoopFilter -> Init : [En == 0]
  ClosedLoop -> Init [order 1] : [En == 0]
  Init -> Align : [En == 1]
  Align -> Init [order 1] : [En == 0]
  OpenLoop -> Init [order 2] : [En == 0]
  Align -> OpenLoop [order 2] : after(0.5,sec)
  ClosedLoop -> ClosedLoopFilter [order 2] : after(0.1,sec)
  OpenLoop -> ClosedLoop [order 1] : after(4,sec)[SpeedFb > Limit]
  data: Limit input fixdt(1,16,14); SpeedFb input fixdt(1,16,14); Mode output uint16; En input boolean; SpeedCtrl output uint16
